simulink model "Sim_singleDOF"  (R2019b)
settings: Solver=FixedStepAuto  StartTime=0.0  StopTime=t_end  FixedStep=0.0002  RelTol=1e-3  EnableMultiTasking=on
values from neighbouring files (symbols this model uses):
  den_Cfb = [0.00109873559912302  1  0]    [main_P_GDIFFT.m]
  den_P = [mass 0 0]    [main_P_GDIFFT.m]
  num_Cfb = [179824.76349148  33696607.3425078  876981355.154548]    [main_P_GDIFFT.m]
  num_P = [1]    [main_P_GDIFFT.m]
settings Model: Creator=SONG  LastModifiedBy=xiaoshu
settings DataIOCC: LimitDataPoints=on  ReturnWorkspaceOutputs=off
settings OptimizationCC: LifeSpan=inf
settings DebuggingCC: AllowSymbolicDim=off  SFUnexpectedBacktrackingDiag=warning  SFNoUnconditionalDefaultTransitionDiag=warning  SFExecutionAtInitializationDiag=none  ArithmeticOperatorsInVariantConditions=warning
settings ModelReferenceCC: PropagateSignalLabelsOutOfModel=off
settings SFSimCC: SimUseLocalCustomCode=off  CustomCodeUndefinedFunction=UseInterfaceOnly
settings RTWCC: RTWUseLocalCustomCode=off
settings CodeAppCC: StateflowObjectComments=on
settings GRTTargetCC: TargetLangStandard=C89/C90 (ANSI)
settings ConfigComp: CovMetricSettings=dw  CovHtmlReporting=on  CovSaveCumulativeToWorkspaceVar=on  CovSaveSingleToWorkspaceVar=on  CovExternalEMLEnable=off

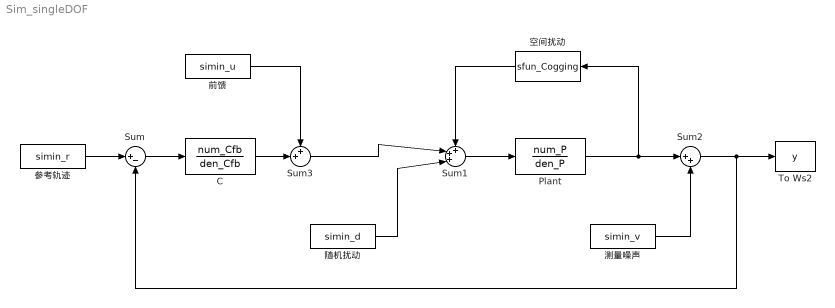
== system Sim_singleDOF ==
  C : TransferFcn  Numerator=num_Cfb  Denominator=den_Cfb
  Plant : TransferFcn  Numerator=num_P  Denominator=den_P
  Sum : Sum  Inputs=|+-
  Sum1 : Sum  Inputs=+++|
  Sum2 : Sum  Inputs=|++
  Sum3 : Sum  Inputs=++|
  To Ws2 : ToWorkspace  VariableName=y  SampleTime=-1
  前馈 : FromWorkspace  VariableName=simin_u  SampleTime=0
  参考轨迹 : FromWorkspace  VariableName=simin_r  SampleTime=0
  测量噪声 : FromWorkspace  VariableName=simin_v  SampleTime=0
  空间扰动 : S-Function  FunctionName=sfun_Cogging  SFunctionDeploymentMode=off  EnableBusSupport=off
  随机扰动 : FromWorkspace  VariableName=simin_d  SampleTime=0
  wires:
  Sum2/1 -> Sum/2, To Ws2/1
  参考轨迹/1 -> Sum/1
  测量噪声/1 -> Sum2/2
  Sum/1 -> C/1
  Sum1/1 -> Plant/1
  空间扰动/1 -> Sum1/1
  Sum3/1 -> Sum1/2
  C/1 -> Sum3/2
  前馈/1 -> Sum3/1
  随机扰动/1 -> Sum1/3
  Plant/1 -> 空间扰动/1, Sum2/1
